simulink model "Registration_Estimation"  (R2016a)
settings: Solver=ode4  StartTime=0.0  StopTime=inf  FixedStep=ts  RelTol=1e-3
undefined symbols (not defined in the file or in its folder): ts
libraries: slrtlib x8, xpcmeasurementcomputinglib x4, xpcconteclib x3, xpcutilitieslib x1, xpcrtudplib x1
settings Model: SimulationMode=external  Creator=Biorobotics  LastModifiedBy=Biorobotics
settings SolverCC: EnableConcurrentExecution=on
settings DataIOCC: SaveFormat=StructureWithTime
settings OptimizationCC: BlockReduction=off  OptimizeBlockIOStorage=off  BufferReuse=off  GlobalBufferReuse=off  ExpressionFolding=off  LocalBlockOutputs=off
settings HardwareCC: ProdBitPerPointer=32  ProdLargestAtomicFloat=None  ProdWordSize=32  ProdLongLongMode=on  ProdHWDeviceType=Generic->32-bit x86 compatible
settings RTWCC: SystemTargetFile=slrt.tlc  TemplateMakefile=slrt_default_tmf  Description=Simulink Real-Time  RTWCompilerOptimization=on

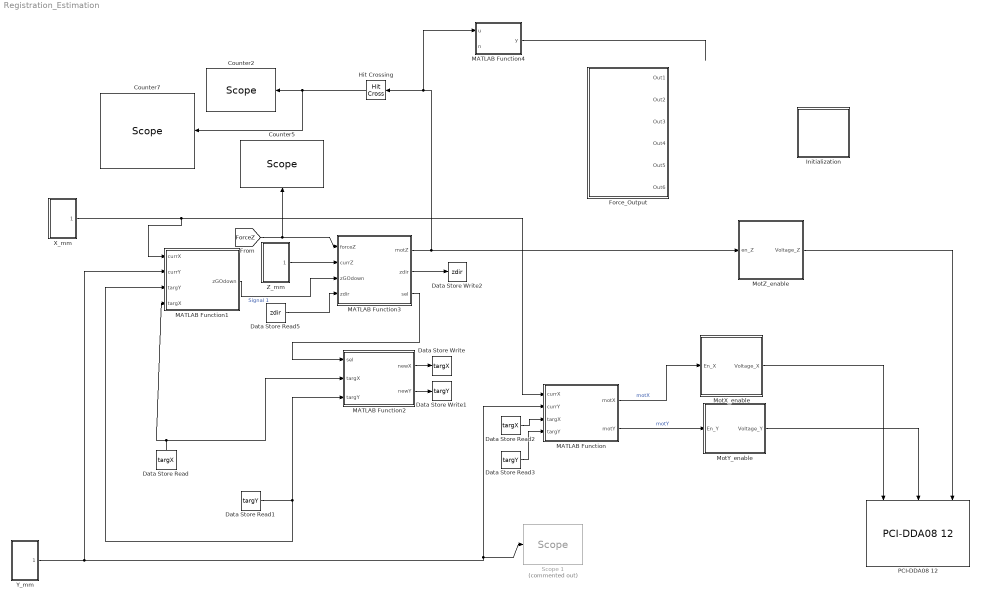
== system Registration_Estimation ==
  Counter2 : slrtlib/Displays and Logging/Scope   scopeno=5  scopetype=Target  autostart=on  viewmode=Graphical rolling  formatstr='%15.6f'  grid=on  ylimits=[0,0]  nosamples=500  noprepostsamples=0  interleave=1  triggermode=FreeRun  triggersignal=1  trigsignalfromport=off  triggerlevel=0.0  triggerslope=Either  triggerscope=1  triggersample=0  filename=data.dat  mode=Lazy  writesize=512  autorestart=off  dynamicfilemode=off  maxwritefilesize=512*1024^2
  Counter5 : slrtlib/Displays and Logging/Scope   scopeno=2  scopetype=Target  autostart=on  viewmode=Numerical  formatstr='%15.6f'  grid=on  ylimits=[0,0]  nosamples=3  noprepostsamples=0  interleave=1  triggermode=FreeRun  triggersignal=1  trigsignalfromport=off  triggerlevel=0.0  triggerslope=Either  triggerscope=1  triggersample=0  filename=data.dat  mode=Lazy  writesize=512  autorestart=off  dynamicfilemode=off  maxwritefilesize=512*1024^2
  Counter7 : slrtlib/Displays and Logging/Scope   scopeno=8  scopetype=File  autostart=on  viewmode=Graphical rolling  formatstr='%15.6f'  grid=on  ylimits=[0,0]  nosamples=500000  noprepostsamples=0  interleave=1  triggermode=FreeRun  triggersignal=1  trigsignalfromport=off  triggerlevel=0.0  triggerslope=Either  triggerscope=1  triggersample=0  filename=enable.dat  mode=Lazy  writesize=512  autorestart=off  dynamicfilemode=off  maxwritefilesize=512*1024^2
  Data Store Read : DataStoreRead  DataStoreName=targX  DataStoreElements=targX
  Data Store Read1 : DataStoreRead  DataStoreName=targY  DataStoreElements=targY
  Data Store Read2 : DataStoreRead  DataStoreName=targX  DataStoreElements=targX
  Data Store Read3 : DataStoreRead  DataStoreName=targY  DataStoreElements=targY
  Data Store Read5 : DataStoreRead  DataStoreName=zdir  DataStoreElements=zdir
  Data Store Write : DataStoreWrite  DataStoreName=targX  DataStoreElements=targX
  Data Store Write1 : DataStoreWrite  DataStoreName=targY  DataStoreElements=targY
  Data Store Write2 : DataStoreWrite  DataStoreName=zdir  DataStoreElements=zdir
  Force_Output : Subsystem
  Hit Crossing : HitCross  HitCrossingDirection=rising
  Initialization : Subsystem
  MATLAB Function : MATLAB Function  TreatAsAtomicUnit=on
  MATLAB Function1 : MATLAB Function  TreatAsAtomicUnit=on
  MATLAB Function2 : MATLAB Function  TreatAsAtomicUnit=on
  MATLAB Function3 : MATLAB Function  TreatAsAtomicUnit=on
  MATLAB Function4 : MATLAB Function  TreatAsAtomicUnit=on
  MotX_enable : Subsystem
  MotY_enable : Subsystem
  MotZ_enable : Subsystem
  "PCI-DDA08 12 " : xpcmeasurementcomputinglib/D//A/PCI-DDA08 12   channel=[1 2 3]  range=[-10 -10 -10]  reset=[1]  initValue=[0]  sampletime=ts  pci_dev=-1
  Scope 1 : slrtlib/Displays and Logging/Scope   Commented=on  scopeno=2  scopetype=File  autostart=on  viewmode=Graphical redraw  formatstr='%15.6f'  grid=on  ylimits=[0,0]  nosamples=200000  noprepostsamples=0  interleave=1  triggermode=FreeRun  triggersignal=1  trigsignalfromport=off  triggerlevel=0.0  triggerslope=Either  triggerscope=1  triggersample=0  filename=Ydata.dat  mode=Lazy  writesize=512  autorestart=off  dynamicfilemode=off  maxwritefilesize=512*1024^2
  X_mm : Subsystem
  Y_mm : Subsystem
  Z_mm : Subsystem
  wires:
  Data Store Read/1 -> MATLAB Function2/2(targX), MATLAB Function1/4(targX)
  Data Store Read1/1 -> MATLAB Function2/3(targY), MATLAB Function1/3(targY)
  MATLAB Function2/2(newY) -> Data Store Write1/1
  Data Store Read2/1 -> MATLAB Function/3(targX)
  Data Store Read3/1 -> MATLAB Function/4(targY)
  MATLAB Function1/1(zGOdown) -> MATLAB Function3/3(zGOdown)  "Signal 1"
  MATLAB Function3/1(motZ) -> MATLAB Function4/1(u), Hit Crossing/1, MotZ_enable/1(en_Z)
  Data Store Read5/1 -> MATLAB Function3/4("zdir ")
  MATLAB Function3/2(zdir) -> Data Store Write2/1
  MATLAB Function3/3(sel) -> MATLAB Function2/1(sel)
  [ForceZ] -> MATLAB Function3/1(forceZ), Counter5/1
  Hit Crossing/1 -> Counter2/1, Counter7/1
  X_mm/1(X_mm) -> MATLAB Function1/1(currX), MATLAB Function/1(currX)
  Y_mm/1(Y_mm) -> MATLAB Function1/2(currY), Scope 1/1, MATLAB Function/2(currY)
  Z_mm/1(Z_mm) -> MATLAB Function3/2(currZ)
  MATLAB Function/1(motX) -> MotX_enable/1(En_X)  "motX"
  MotX_enable/1(Voltage_X) -> "PCI-DDA08 12 "/1
  MATLAB Function/2(motY) -> MotY_enable/1(En_Y)  "motY"
  MotY_enable/1(Voltage_Y) -> "PCI-DDA08 12 "/2
  MotZ_enable/1(Voltage_Z) -> "PCI-DDA08 12 "/3
  MATLAB Function2/1(newX) -> Data Store Write/1
  MATLAB Function4/1(y) -> ?

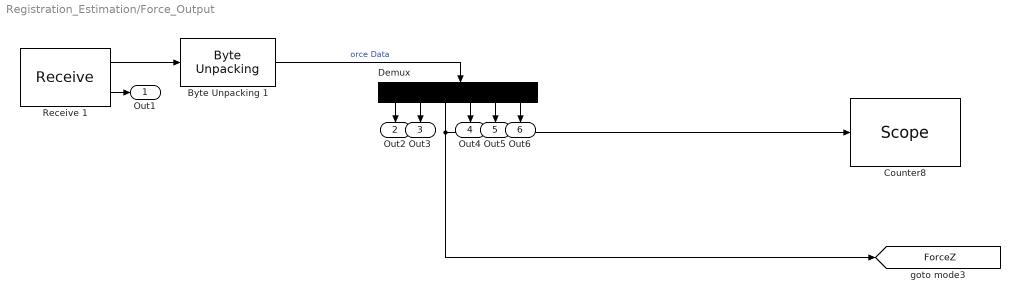
== system Registration_Estimation/Force_Output ==
  Byte Unpacking 1 : xpcutilitieslib/Byte Unpacking   MaskUnpackedDataTypes={'double'}  MaskUnpackedDataSizes={[6]}  MaskAlignment=1
  Counter8 : slrtlib/Displays and Logging/Scope   scopeno=9  scopetype=Target  autostart=on  viewmode=Graphical rolling  formatstr='%15.6f'  grid=on  ylimits=[0,0]  nosamples=2000  noprepostsamples=0  interleave=1  triggermode=FreeRun  triggersignal=1  trigsignalfromport=off  triggerlevel=0.0  triggerslope=Either  triggerscope=1  triggersample=0  filename=data.dat  mode=Lazy  writesize=512  autorestart=off  dynamicfilemode=off  maxwritefilesize=512*1024^2
  Demux : Demux  Outputs=6
  Receive 1 : xpcrtudplib/Legacy UDP/Receive   ipAddress=192.168.1.2  ipPort=25000  width=48  vblLen=off  sampletime=ts
  Out1 : Outport
  Out2 : Outport  Port=2
  Out3 : Outport  Port=3
  Out4 : Outport  Port=4
  Out5 : Outport  Port=5
  Out6 : Outport  Port=6
  tag scope: ForceZ=global
  wires:
  Byte Unpacking 1/1 -> Demux/1  "orce Data"
  Receive 1/1 -> Byte Unpacking 1/1
  Demux/3 -> [ForceZ], Counter8/1
  Demux/6 -> Out6/1
  Demux/2 -> Out3/1
  Demux/5 -> Out5/1
  Receive 1/2 -> Out1/1
  Demux/4 -> Out4/1
  Demux/1 -> Out2/1

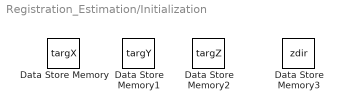
== system Registration_Estimation/Initialization ==
  Data Store Memory : DataStoreMemory  DataStoreName=targX  ReadBeforeWriteMsg=warning  WriteAfterWriteMsg=warning  WriteAfterReadMsg=warning  InitialValue=40  ShowAdditionalParam=off
  Data Store Memory1 : DataStoreMemory  DataStoreName=targY  ReadBeforeWriteMsg=warning  WriteAfterWriteMsg=warning  WriteAfterReadMsg=warning  InitialValue=40  ShowAdditionalParam=off
  Data Store Memory2 : DataStoreMemory  DataStoreName=targZ  ReadBeforeWriteMsg=warning  WriteAfterWriteMsg=warning  WriteAfterReadMsg=warning  InitialValue=20  ShowAdditionalParam=off
  Data Store Memory3 : DataStoreMemory  DataStoreName=zdir  ReadBeforeWriteMsg=warning  WriteAfterWriteMsg=warning  WriteAfterReadMsg=warning  InitialValue=-1  ShowAdditionalParam=off

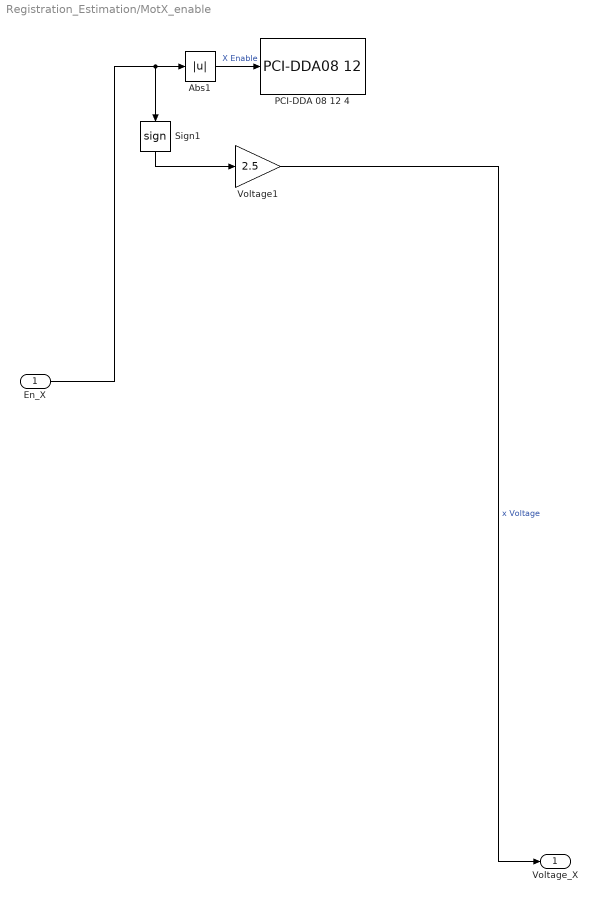
== system Registration_Estimation/MotX_enable ==
  En_X : Inport
  Abs1 : Abs
  PCI-DDA 08 12 4 : xpcmeasurementcomputinglib/Digital Output/PCI-DDA08 12   channel=1  port=A  reset=[1]  initValue=[0]  chip=1  sampletime=ts  slot=-1
  Sign1 : Signum
  Voltage1 : Gain  Gain=2.5
  Voltage_X : Outport
  wires:
  Sign1/1 -> Voltage1/1
  En_X/1 -> Abs1/1, Sign1/1
  Abs1/1 -> PCI-DDA 08 12 4/1  "X Enable"
  Voltage1/1 -> Voltage_X/1  "x Voltage"

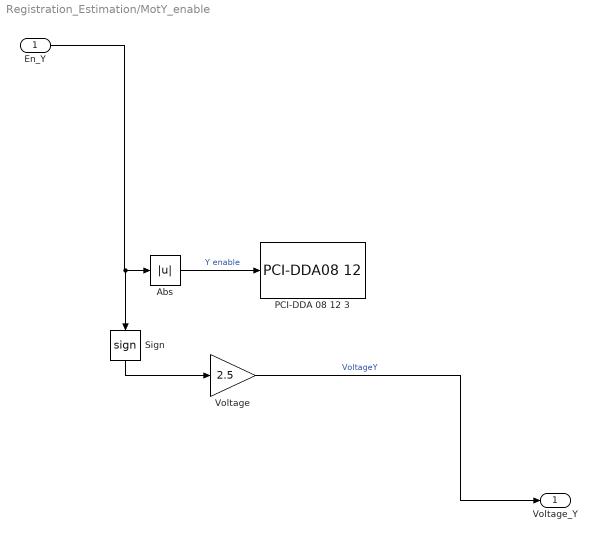
== system Registration_Estimation/MotY_enable ==
  En_Y : Inport
  Abs : Abs
  PCI-DDA 08 12 3 : xpcmeasurementcomputinglib/Digital Output/PCI-DDA08 12   channel=3  port=A  reset=[1]  initValue=[0]  chip=1  sampletime=ts  slot=-1
  Sign : Signum
  Voltage : Gain  Gain=2.5
  Voltage_Y : Outport
  wires:
  Abs/1 -> PCI-DDA 08 12 3/1  "Y enable"
  Sign/1 -> Voltage/1
  Voltage/1 -> Voltage_Y/1  "VoltageY"
  En_Y/1 -> Sign/1, Abs/1

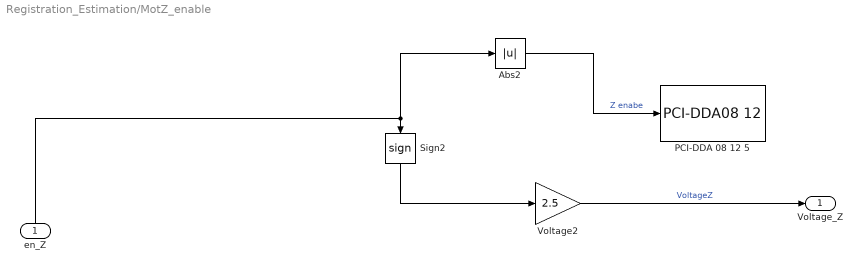
== system Registration_Estimation/MotZ_enable ==
  en_Z : Inport
  Abs2 : Abs
  PCI-DDA 08 12 5 : xpcmeasurementcomputinglib/Digital Output/PCI-DDA08 12   channel=5  port=A  reset=[1]  initValue=[0]  chip=1  sampletime=ts  slot=-1
  Sign2 : Signum
  Voltage2 : Gain  Gain=2.5
  Voltage_Z : Outport
  wires:
  en_Z/1 -> Abs2/1, Sign2/1
  Abs2/1 -> PCI-DDA 08 12 5/1  "Z enabe"
  Sign2/1 -> Voltage2/1
  Voltage2/1 -> Voltage_Z/1  "VoltageZ"

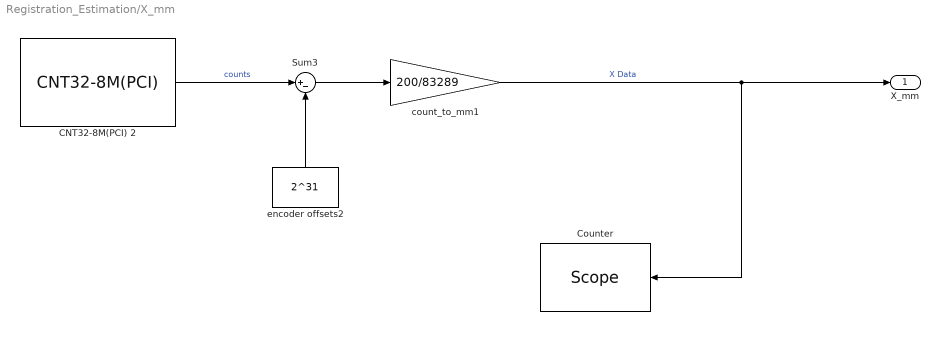
== system Registration_Estimation/X_mm ==
  CNT32-8M(PCI) 2 : xpcconteclib/Incremental Encoder/CNT32-8M(PCI)   Channel=1  OperationMode=2-phase Input Synchronous Clear Multiply by 4  DigitalFilter=No filtering  PulseInput=TTL level input  Direction=Up in the clockwise direction/Down in the counterclockwise direction  InitialValue=2^31  LoadInitialValue=on  SampleTime=ts  PciSlot=[4 5]  StartMethod=Model Start  StopMethod=Model Terminate  ZeroClearRising=off  ZeroClearFalling=off  ZeroClearMatch0=off  ZeroClearMatch1=off  PresetRising=off  PresetFalling=off  PresetMatch0=off  PresetMatch1=off  PresetValue=0  Match0Value=0  Match1Value=0  OutputSignalMatch0=off  OutputSignalMatch1=off  OutputSignalAbnormal=off  OutputSignalDigitalFilter=off  OutputSignalAlarm=off  OneShotDuration=10 microseconds  IndexEnable=Disable  IndexLogic=Positive (Active High)  EnableDigitalInput=off  EnableDigitalOutput=off  DigitalOutputInitialValue=None  DigitalOutputFinalValue=None
  Counter : slrtlib/Displays and Logging/Scope   scopeno=3  scopetype=File  autostart=on  viewmode=Numerical  formatstr='%15.6f'  grid=on  ylimits=[0,0]  nosamples=500000  noprepostsamples=0  interleave=1  triggermode=FreeRun  triggersignal=1  trigsignalfromport=off  triggerlevel=0.0  triggerslope=Either  triggerscope=1  triggersample=0  filename=Xdata.dat  mode=Lazy  writesize=512  autorestart=off  dynamicfilemode=off  maxwritefilesize=512*1024^2
  Sum3 : Sum  Inputs=|+-
  count_to_mm1 : Gain  Gain=200/83289
  encoder offsets2 : Constant  Value=2^31
  X_mm : Outport
  wires:
  encoder offsets2/1 -> Sum3/2
  CNT32-8M(PCI) 2/1 -> Sum3/1  "counts"
  Sum3/1 -> count_to_mm1/1
  count_to_mm1/1 -> Counter/1, X_mm/1  "X Data"

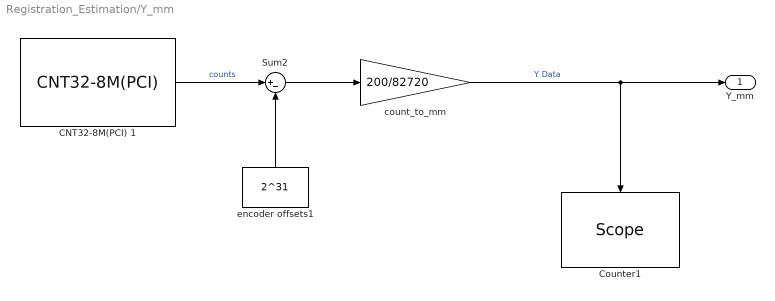
== system Registration_Estimation/Y_mm ==
  CNT32-8M(PCI) 1 : xpcconteclib/Incremental Encoder/CNT32-8M(PCI)   Channel=2  OperationMode=2-phase Input Synchronous Clear Multiply by 4  DigitalFilter=No filtering  PulseInput=TTL level input  Direction=Up in the clockwise direction/Down in the counterclockwise direction  InitialValue=2^31  LoadInitialValue=on  SampleTime=ts  PciSlot=[4 5]  StartMethod=Model Start  StopMethod=Model Terminate  ZeroClearRising=off  ZeroClearFalling=off  ZeroClearMatch0=off  ZeroClearMatch1=off  PresetRising=off  PresetFalling=off  PresetMatch0=off  PresetMatch1=off  PresetValue=0  Match0Value=0  Match1Value=0  OutputSignalMatch0=off  OutputSignalMatch1=off  OutputSignalAbnormal=off  OutputSignalDigitalFilter=off  OutputSignalAlarm=off  OneShotDuration=10 microseconds  IndexEnable=Disable  IndexLogic=Positive (Active High)  EnableDigitalInput=off  EnableDigitalOutput=off  DigitalOutputInitialValue=None  DigitalOutputFinalValue=None
  Counter1 : slrtlib/Displays and Logging/Scope   scopeno=4  scopetype=File  autostart=on  viewmode=Numerical  formatstr='%15.6f'  grid=on  ylimits=[0,0]  nosamples=500000  noprepostsamples=0  interleave=1  triggermode=FreeRun  triggersignal=1  trigsignalfromport=off  triggerlevel=0.0  triggerslope=Either  triggerscope=1  triggersample=0  filename=Ydata.dat  mode=Lazy  writesize=512  autorestart=off  dynamicfilemode=off  maxwritefilesize=512*1024^2
  Sum2 : Sum  Inputs=|+-
  count_to_mm : Gain  Gain=200/82720
  encoder offsets1 : Constant  Value=2^31
  Y_mm : Outport
  wires:
  encoder offsets1/1 -> Sum2/2
  CNT32-8M(PCI) 1/1 -> Sum2/1  "counts"
  Sum2/1 -> count_to_mm/1
  count_to_mm/1 -> Y_mm/1, Counter1/1  "Y Data"

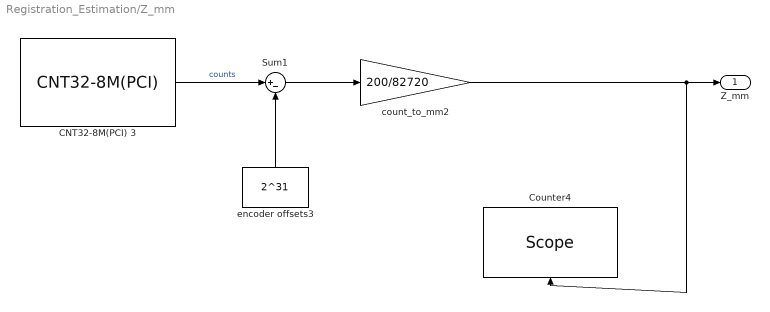
== system Registration_Estimation/Z_mm ==
  CNT32-8M(PCI) 3 : xpcconteclib/Incremental Encoder/CNT32-8M(PCI)   Channel=4  OperationMode=2-phase Input Synchronous Clear Multiply by 4  DigitalFilter=No filtering  PulseInput=TTL level input  Direction=Up in the clockwise direction/Down in the counterclockwise direction  InitialValue=2^31  LoadInitialValue=on  SampleTime=ts  PciSlot=[4 5]  StartMethod=Model Start  StopMethod=Model Terminate  ZeroClearRising=off  ZeroClearFalling=off  ZeroClearMatch0=off  ZeroClearMatch1=off  PresetRising=off  PresetFalling=off  PresetMatch0=off  PresetMatch1=off  PresetValue=0  Match0Value=0  Match1Value=0  OutputSignalMatch0=off  OutputSignalMatch1=off  OutputSignalAbnormal=off  OutputSignalDigitalFilter=off  OutputSignalAlarm=off  OneShotDuration=10 microseconds  IndexEnable=Disable  IndexLogic=Positive (Active High)  EnableDigitalInput=off  EnableDigitalOutput=off  DigitalOutputInitialValue=None  DigitalOutputFinalValue=None
  Counter4 : slrtlib/Displays and Logging/Scope   scopeno=1  scopetype=File  autostart=on  viewmode=Numerical  formatstr='%15.6f'  grid=on  ylimits=[0,0]  nosamples=500000  noprepostsamples=0  interleave=1  triggermode=FreeRun  triggersignal=1  trigsignalfromport=off  triggerlevel=0.0  triggerslope=Either  triggerscope=1  triggersample=0  filename=Zdata.dat  mode=Lazy  writesize=512  autorestart=off  dynamicfilemode=off  maxwritefilesize=512*1024^2
  Sum1 : Sum  Inputs=|+-
  count_to_mm2 : Gain  Gain=200/82720
  encoder offsets3 : Constant  Value=2^31
  Z_mm : Outport
  wires:
  count_to_mm2/1 -> Counter4/1, Z_mm/1
  CNT32-8M(PCI) 3/1 -> Sum1/1  "counts"
  Sum1/1 -> count_to_mm2/1
  encoder offsets3/1 -> Sum1/2

== matlab function Registration_Estimation/MATLAB Function1 ==
  data: currX input; zGOdown output; currY input; targY input; targX input
function zGOdown  = PosReach(currX,currY,targY,targX)
%#codegen
    currX = ceil(currX);
    currY = ceil(currY);
    targX = ceil(targX);
    targY = ceil(targY);
    
    
    if((currX==targX)&&(currY==targY))
       	zGOdown = 1; %if target position reached 
    else
        zGOdown = 0; %otherwise
    end
end

== matlab function Registration_Estimation/MATLAB Function ==
  data: currX input; motX output; currY input; motY output; targX input; targY input
function [motX,motY] = moveMot (currX,currY,targX,targY)
%#codegen
%#codegen
motX=0;
motY=0;
currX = ceil(currX);
currY = ceil(currY);
targX = ceil(targX);
targY = ceil(targY);

if(targX>currX)
    motX=-1;
end
if(targX<currX)
    motX=+1;
end
if(targY>currY)
    motY=-1;
end
if(targY<currY)
    motY=1;
end


end

== matlab function Registration_Estimation/MATLAB Function2 ==
  data: sel input; newX output; targX input; targY input; newY output
function [newX,newY] = genXY(sel,targX,targY)
%#codegen

    if(sel ==0)
        newX=targX;
        newY=targY;
    else
       newX = -5+70*rand;
       newY = -5+70*rand;%gerenrate random num
%         newX = 5;
%         newY = 5;
    end
end

== matlab function Registration_Estimation/MATLAB Function3 ==
  data: forceZ input; currZ input; zGOdown input; motZ output; zdir output; zdir input; sel output
function [motZ,zdir,sel] = Zdown(forceZ,currZ,zGOdown,zdir)
%#codegen
motZ = 0;
currZ = ceil(currZ);
sel=0;
temp = zdir;
fthresh=0.0075;
if((forceZ > -fthresh)&&(zGOdown==1)&&(zdir==-1))
    % Force is less and XY have reached and direction is down
    motZ = -1; %Move motor down
    
elseif((currZ >=0)&&(zGOdown==1)&&(zdir==1))
    % If Z is higher and XY reached and direction is up
    motZ = 1; %move motor up
    
elseif(forceZ<=-fthresh)
    % Force exceeds on organ so move up
    zdir=1;
end

% If prev direction is up and currently Z is lower
if((temp==1)&&(currZ<=0))
    
    sel=1;
    zdir = -1;
end
end

== matlab function Registration_Estimation/MATLAB Function4 ==
  data: u input; y output; n input
function y = fcn(u,n)
%#codegen

y = u;
